simulink model "PID_Compensacion_De_Gravedad"  (R2021b)
settings: Solver=VariableStepAuto  StartTime=0.0  StopTime=20  RelTol=1e-3
settings Model: Creator=Marco  LastModifiedBy=Marco

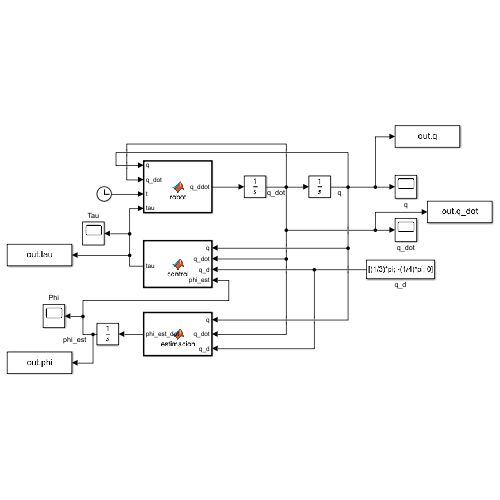
[thumbnail: Simulink's stored preview of the top-level diagram]
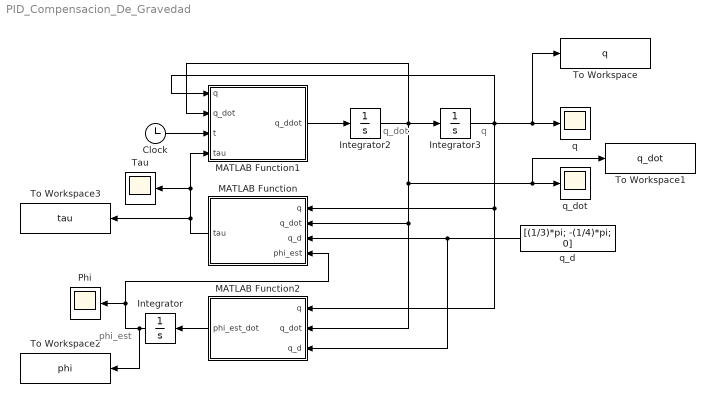
== system PID_Compensacion_De_Gravedad ==
  note: phi_est
  note: q
  note: q_dot
  Clock : Clock
  Integrator : Integrator
  Integrator2 : Integrator  InitialCondition=[0; 0; 0]
  Integrator3 : Integrator  InitialCondition=[0; 0; 0]
  MATLAB Function : MATLAB Function  TreatAsAtomicUnit=on
  MATLAB Function1 : MATLAB Function  TreatAsAtomicUnit=on
  MATLAB Function2 : MATLAB Function  TreatAsAtomicUnit=on
  Phi : Scope
  Tau : Scope
  To Workspace : ToWorkspace  VariableName=q  SaveFormat=Timeseries  SampleTime=-1
  To Workspace1 : ToWorkspace  VariableName=q_dot  SaveFormat=Timeseries  SampleTime=-1
  To Workspace2 : ToWorkspace  VariableName=phi  SaveFormat=Timeseries  SampleTime=-1
  To Workspace3 : ToWorkspace  VariableName=tau  SaveFormat=Timeseries  SampleTime=-1
  q : Scope
  q_d : Constant  Value=[(1/3)*pi; -(1/4)*pi; 0]
  q_dot : Scope
  wires:
  Integrator3/1 -> MATLAB Function2/1(q), MATLAB Function/1(q), To Workspace/1, q/1, MATLAB Function1/1(q)
  MATLAB Function1/1(q_ddot) -> Integrator2/1
  MATLAB Function/1(tau) -> To Workspace3/1, MATLAB Function1/4(tau), Tau/1
  MATLAB Function2/1(phi_est_dot) -> Integrator/1
  Integrator/1 -> To Workspace2/1, Phi/1, MATLAB Function/4(phi_est)
  q_d/1 -> MATLAB Function2/3(q_d), MATLAB Function/3(q_d)
  Integrator2/1 -> MATLAB Function2/2(q_dot), MATLAB Function/2(q_dot), To Workspace1/1, q_dot/1, MATLAB Function1/2(q_dot), Integrator3/1
  Clock/1 -> MATLAB Function1/3(t)

== matlab function PID_Compensacion_De_Gravedad/MATLAB Function1 ==
  data: q input; q_dot input; t input; q_ddot output; tau input
function q_ddot = robot(q, q_dot, t, tau)
%Parametros fisicos del robot
g = 9.81;
l_1 = 0.26;
l_2 = 0.26;
l_3 = 0.26;
lc_1 = 0.0983;
lc_2 = 0.0229;
lc_3 = 0.0229;
m_1 = 6.5225;
m_2 = 2.0458;

if t > 10
    m_3 = 4;
else
    m_3 = 2.0458;
end

I_1 = 0.1213;
I_2 = 0.0616;
I_3 = 0.0616;
                                                                                                                              %
%Constantes
phi_1 = m_1*lc_1^2 + I_1 + m_2*l_1^2 + m_2*lc_2^2 + I_2 + m_3*l_1^2 + m_3*l_2^2 + m_3*lc_3^2 + I_3;
phi_2 = m_2*l_1*lc_2 + m_3*l_1*l_2;
phi_3 = m_3*l_2*lc_3;
phi_4 = m_3*l_1*lc_3;
phi_5 = m_2*lc_2^2 + I_2 + m_3*l_2^2 + m_3*lc_3^2 + I_3;
phi_6 = m_3*lc_3^2 + I_3;
phi_7 = m_1*lc_1 + (m_2 + m_3)*l_1;
phi_8 = m_2*lc_2 + m_3*l_2;
phi_9 = m_3*lc_3;
phi = [phi_1; phi_2; phi_3; phi_4; phi_5; phi_6; phi_7; phi_8; phi_9];

%Matriz de inercia M(q)
m_11 = phi(1) + 2*phi(2)*cos(q(2)) + 2*phi(3)*cos(q(3)) + 2*phi(4)*cos(q(2)+q(3));
m_12 = phi(5) + phi(2)*cos(q(2)) + 2*phi(3)*cos(q(3)) + phi(4)*cos(q(2)+q(3));
m_13 = phi(6) + phi(3)*cos(q(3)) + phi(4)*cos(q(2)+q(3));
m_21 = m_12;
m_22 = phi(5) + 2*phi(3)*cos(q(3));
m_23 = phi(6) + phi(3)*cos(q(3));
m_31 = m_13;
m_32 = m_23;
m_33 = phi(6);

M = [m_11 m_12 m_13;
     m_21 m_22 m_23;
     m_31 m_32 m_33];

%Matriz de Coriolis C(q,qd)
c_11 = -phi(2)*sin(q(2))*q_dot(2) - phi(3)*sin(q(3))*q_dot(3) - phi(4)*sin(q(2)+q(3))*(q_dot(2)+q_dot(3));
c_12 = -phi(2)*sin(q(2))*(q_dot(1)+q_dot(2)) - phi(3)*sin(q(3))*q_dot(3) - phi(4)*sin(q(2)+q(3))*(q_dot(1)+q_dot(2)+q_dot(3));
c_13 = -phi(3)*sin(q(3))*(q_dot(1)+q_dot(2)+q_dot(3)) - phi(4)*sin(q(2)+q(3))*(q_dot(1)+q_dot(2)+q_dot(3));
c_21 = phi(2)*sin(q(2))*q_dot(1) - phi(3)*sin(q(3))*q_dot(3) + phi(4)*sin(q(2)+q(3))*q_dot(1);
c_22 = -phi(3)*sin(q(3))*q_dot(3);
c_23 = -phi(3)*sin(q(3))*(q_dot(1)+q_dot(2)+q_dot(3));
c_31 = phi(3)*sin(q(3))*(q_dot(1)+q_dot(2)) + phi(4)*sin(q(2)+q(3))*q_dot(1);
c_32 = phi(3)*sin(q(3))*(q_dot(1)+q_dot(2));
c_33 = 0;

C = [c_11 c_12 c_13;
     c_21 c_22 c_23;
     c_31 c_32 c_33];

%Vector de gravedad g(q)
g_1 = g*phi(7)*cos(q(1)) + g*phi(8)*cos(q(1)+q(2)) + g*phi(9)*cos(q(1)+q(2)+q(3));
g_2 = g*phi(8)*cos(q(1)+q(2)) + g*phi(9)*cos(q(1)+q(2)+q(3));
g_3 = g*phi(9)*cos(q(1)+q(2)+q(3));

G = [g_1;
     g_2;
     g_3];

%Dinamica del manipulador
q_ddot = - inv(M)*(C*q_dot + G - tau);

end

== matlab function PID_Compensacion_De_Gravedad/MATLAB Function ==
  data: q input; q_dot input; q_d input; tau output; phi_est input
function tau = control(q, q_dot, q_d, phi_est)
%Gravedad y ganancias
g = 9.81;

p = 15;
d = 8; 

%Regresor Y_G
Y_G = zeros(3,9);

Y_G(1,7) = g*cos(q(1));
Y_G(1,8) = g*cos(q(1)+q(2));
Y_G(1,9) = g*cos(q(1)+q(2)+q(3));
Y_G(2,8) = g*cos(q(1)+q(2));
Y_G(2,9) = g*cos(q(1)+q(2)+q(3));
Y_G(3,9) = g*cos(q(1)+q(2)+q(3));

%Control
tau = -p*(q - q_d) - d*q_dot + Y_G*phi_est;

end

== matlab function PID_Compensacion_De_Gravedad/MATLAB Function2 ==
  data: q input; phi_est_dot output; q_dot input; q_d input
function phi_est_dot  = estimacion(q, q_dot, q_d)
%Gravedad y ganancias
g = 9.81;
 
k = 5;
gamma = 1;

%Regresor Y_G
Y_G = zeros(3,9);

Y_G(1,7) = g*cos(q(1));
Y_G(1,8) = g*cos(q(1)+q(2));
Y_G(1,9) = g*cos(q(1)+q(2)+q(3));
Y_G(2,8) = g*cos(q(1)+q(2));
Y_G(2,9) = g*cos(q(1)+q(2)+q(3));
Y_G(3,9) = g*cos(q(1)+q(2)+q(3));

%Ley De Estimacion 

q_e = q - q_d;

phi_est_dot = -k*Y_G'*(q_dot + gamma*(1/(1 + q_e'*q_e))*q_e);

end
